simulink model "meranie_prevodovej_charakteristiky"  (R2019b)
settings: Solver=VariableStepAuto  StartTime=0.0  StopTime=100  RelTol=1e-3
values from neighbouring files (symbols this model uses):
  beta = 0.5*sqrt(g/l)    [cv_3.m]    (also in prev_char.m)
  g = 9.81    [cv_3.m]    (also in prev_char.m)
  l = 1    [cv_3.m]    (also in prev_char.m)
  m = 1    [cv_3.m]    (also in prev_char.m)
  Ts = 0.1    [cv_3.m]    (also in prev_char.m)
libraries: simulink x2
settings Model: Creator=Martin Dodek  LastModifiedBy=Martin Dodek

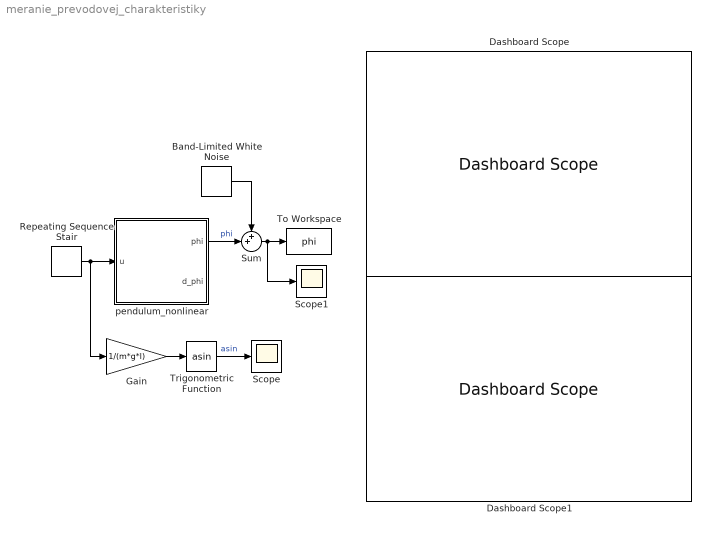
== system meranie_prevodovej_charakteristiky ==
  Band-Limited White Noise : simulink/Sources/Band-Limited White Noise  Cov=1e-6  Ts=Ts  seed=[23341]
  Dashboard Scope : DashboardScope
  Dashboard Scope1 : DashboardScope
  Gain : Gain  Gain=1/(m*g*l)
  Repeating Sequence Stair : simulink/Sources/Repeating Sequence Stair  OutValues=[0:1:9]  tsamp=10  OutMin=[]  OutMax=[]  OutDataTypeStr=double  OutputDataTypeScalingMode=double  OutDataType=fixdt(0,8)  ConRadixGroup=Best Precision: Vector-wise  OutScaling=2^-12
  Scope : Scope
  Scope1 : Scope
  Sum : Sum  Inputs=++|
  To Workspace : ToWorkspace  VariableName=phi  SampleTime=-1
  Trigonometric Function : Trigonometry  Operator=asin
  pendulum_nonlinear : Subsystem
  wires:
  pendulum_nonlinear/1(phi) -> Sum/2  "phi"
  Band-Limited White Noise/1 -> Sum/1
  Repeating Sequence Stair/1 -> Gain/1, pendulum_nonlinear/1(u)
  Trigonometric Function/1 -> Scope/1  "asin"
  Gain/1 -> Trigonometric Function/1
  Sum/1 -> Scope1/1, To Workspace/1

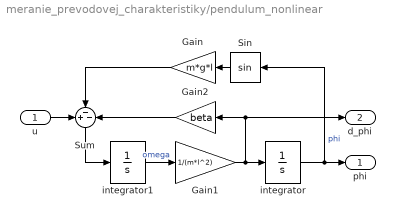
== system meranie_prevodovej_charakteristiky/pendulum_nonlinear ==
  u : Inport
  Gain : Gain  Gain=m*g*l
  Gain1 : Gain  Gain=1/(m*l^2)
  Gain2 : Gain  Gain=beta
  Sin : Trigonometry
  Sum : Sum  Inputs=+--
  integrator : Integrator
  integrator1 : Integrator
  phi : Outport
  d_phi : Outport  Port=2
  wires:
  integrator/1 -> phi/1, Sin/1  "phi"
  integrator1/1 -> Gain1/1  "omega"
  Sin/1 -> Gain/1
  Gain1/1 -> d_phi/1, Gain2/1, integrator/1
  Sum/1 -> integrator1/1
  u/1 -> Sum/1
  Gain2/1 -> Sum/3
  Gain/1 -> Sum/2
